simulink model "rtwdemo_pmsmfoc_system_nn"  (Simulink 7.9)
settings: Solver=ode45  SolverMode=SingleTasking  StartTime=0.0  StopTime=0.2  FixedStep=40e-6  RelTol=1e-3
PreLoadFcn:
  | rtwdemo_pmsmfoc_data
StartFcn:
  | clear executionProfile
StopFcn:
  | try
  |   AddExecutionProfileToDataInspector();
  | end
undefined symbols (not defined in the file or in its folder): ctrlConst, DiscIntNeverNeededParam, EnumCommandType, pmsm, sensors, sigbuilder_block
libraries: powerlib x7, simulink x2
Description:
  | Field-Oriented Control of Permanent Magnet Synchronous Machine
  | 
  | Demonstrates a Field-Oriented Control algorithm with Space Vector Modulation for a Permanent Magnet Synchronous Machine (PMSM).
  | The test bench can be used to evaluate the system performance. Examples include turning the motor on, searching for a valid rotor position,
  | transitioning to closed loop operation, and changing speed and torque during closed loop control.
  | The Embedded Processor subsystem contains the controller algorithm (which supports C code generation) as well as simulation models of peripherals.
settings Model: Creator=The MathWorks Inc.  LastModifiedBy=bas  CovMetricSettings=dcmtrzow  CovHTMLOptions=-aTS=1 -bRG=1 -bTC=1 -hTR=0 -nFC=0 -scm=1 -bcm=1 -xEv=0  CovModelRefEnable=off
settings DataIOCC: SaveOutput=off  SaveTime=off
settings OptimizationCC: InlineParams=on  InlineInvariantSignals=on  EnhancedBackFolding=on  StrengthReduction=on  ZeroExternalMemoryAtStartup=off  EfficientFloat2IntCast=on  OptimizeModelRefInitCode=on  LifeSpan=1
settings DebuggingCC: AlgebraicLoopMsg=none  SolverPrmCheckMsg=none  SingleTaskRateTransMsg=error  IntegerOverflowMsg=none  ParameterPrecisionLossMsg=none  UnconnectedInputMsg=none  UnconnectedOutputMsg=none  UnconnectedLineMsg=none  UniqueDataStoreMsg=error  AssertControl=DisableAll
settings HardwareCC: ProdEndianess=LittleEndian  ProdHWDeviceType=Generic->32-bit Embedded Processor
settings ModelReferenceCC: ModelReferenceNumInstancesAllowed=Single
settings RTWCC: SystemTargetFile=nanonote.tlc  TemplateMakefile=nanonote.tmf  Description=Ben NanoNote  GenerateReport=on  RTWVerbose=off  ProcessScript=nanonote_make_rtw_hook  IncludeHyperlinkInReport=on  GenerateTraceInfo=on  GenerateTraceReport=on  GenerateTraceReportSl=on  GenerateTraceReportSf=on  GenerateTraceReportEml=on
settings CodeAppCC: IgnoreCustomStorageClasses=off  IgnoreTestpoints=on  MaxIdLength=64  MATLABFcnDesc=on  CustomSymbolStrGlobalVar=$N$M  CustomSymbolStrType=$N$M  CustomSymbolStrFcn=$N$M$F  CustomSymbolStrFcnArg=$I$N$M  CustomSymbolStrBlkIO=$N$M  CustomSymbolStrMacro=$N$M  MATLABSourceComments=on
settings STFCustomTargetCC: CodeReplacementLibrary=ANSI_C  CombineOutputUpdateFcns=on  ERTCustomFileBanners=on  SupportContinuousTime=off  SupportNonInlinedSFcns=off  GRTInterface=off  SystemTargetFile=nanonote.tlc
settings ERTTargetCC: CodeReplacementLibrary=ANSI_C  MultiwordLength=2048  ParMdlRefBuildCompliant=off  CompOptLevelCompliant=off  ConcurrentExecutionCompliant=off  ERTFirstTimeCompliant=off  ModelStepFunctionPrototypeControlCompliant=off  CPPClassGenCompliant=off  InlinedParameterPlacement=NonHierarchical  ERTCustomFileTemplate=nanonote_srmain.tlc  ConvertIfToSwitch=off  SuppressUnreachableDefaultCases=off
settings CustomProperty: Value=on

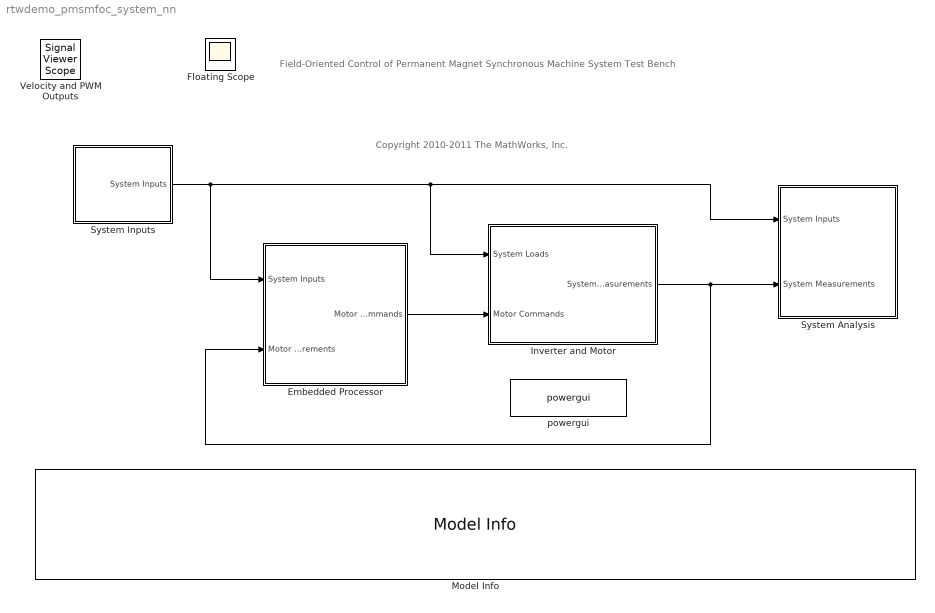
== system rtwdemo_pmsmfoc_system_nn ==
  note: Field-Oriented Control of Permanent Magnet Synchronous Machine
      | System Test Bench
  note: Copyright 2010-2011 The MathWorks, Inc.
  Embedded Processor : Subsystem
      mask Display: image(imread('rtwdemo_pmsmfoc_processor.png'))
  Inverter and Motor : Subsystem  Description=""
      mask Display: image(imread('rtwdemo_pmsmfoc_motor.png'))
  Model Info : simulink/Model-Wide Utilities/Model Info  InitialBlockCM=None  BlockCM=None  Frame=on  DisplayStringWithTags=Model Description: %<Description>  HorizontalTextAlignment=Left  LeftAlignmentValue=0.02  SourceBlockDiagram=rtwdemo_pmsmfoc_system_nn  TagMaxNumber=20
  System Analysis : Subsystem  Description=|
      | System Analysis for Speed Control Design
      | 
      | Analyize and plot signals used to analyize performance of
      | speed  control designs
      mask Display: fprintf('System\nAnalysis')
  System Inputs : Subsystem  Description=""
      mask Display: fprintf('System\nInputs')
  powergui : powerlib/powergui  Priority=1  SimulationMode=Discrete  SolverType=Tustin  SampleTime=1e-005  frequency=60  SPID=off  DisableSnubberDevices=off  DisableRonSwitches=off  DisableVfSwitches=off  SwTol=0  Interpol=off  DisplayEquations=off  FunctionMessages=off  frequencyindice=0  Pbase=100e6  ErrMax=1e-4  Iterations=50  UnitsV=kV  UnitsW=MW  echomessages=off  HookPort=off  EnableUseOfTLC=off  x0status=blocks  RestoreLinks=warning  ResistiveCurrentMeasurement=off  Frange=[0:2:500]  Ylog=off  Xlog=on  ShowGrid=off  save=off  variable=ZData  ZoomFFT=on  StartTime=0.0  cycles=1  DisplayStyle=1  fundamental=60  FreqAxis=off  MaxFrequency=1000  frequencyindicesteady=1  RmsSteady=1  display=off  Ts=0  methode=off
  Floating Scope : Scope
      settings: Floating=on
  Velocity and PWM Outputs : SignalViewerScope  IOType=viewer  NumInputPorts=2  ZoomMode=yonly  RefreshTime=0.035000
      settings: TimeRange=0.14  YMin=-500~0  YMax=4000~3000  SaveName=ScopeData4
  wires:
  Embedded Processor/1(Motor Commands) -> Inverter and Motor/2(Motor Commands)
  Inverter and Motor/1(System Measurements) -> System Analysis/2(System Measurements), Embedded Processor/2(Motor Measurements)
  System Inputs/1(System Inputs) -> System Analysis/1(System Inputs), Inverter and Motor/1(System Loads), Embedded Processor/1(System Inputs)

== system rtwdemo_pmsmfoc_system_nn/Embedded Processor ==
  note: Models hardware on the embedded processor, including
      | the controller algorithm software specification and peripherals.
  note: Embedded Processor
  System Inputs : Inport
  Motor Measurements : Inport  Port=2
  Command Channel : Subsystem  Description=""
      mask Display: fprintf('Command\nChannel')
  Controller Algorithm Software Specification : ModelReference  ModelNameDialog=rtwdemo_pmsmfoc_nn  SimulationMode=Processor-in-the-loop (PIL)  ModelReferenceVersion=1.2950  CopyOfModelName=rtwdemo_pmsmfoc_nn  DefaultDataLogging=on
  Driver Peripherals : Subsystem  Description=""
      mask Display: fprintf('Drivers\nPeripherals')
  Sensor Peripherals : Subsystem  Description=|
      | Elaborate Sensor Models
      | 
      | ADC and QEP and Encoder Models
      mask Display: fprintf('Sensor\nPeripherals')
  Motor Commands : Outport
  wires:
  System Inputs/1 -> Command Channel/1(System Inputs)
  Motor Measurements/1 -> Sensor Peripherals/1(System Measurements)
  Driver Peripherals/1(PWM Duty Cycle) -> Motor Commands/1
  Command Channel/1(motor_on) -> Controller Algorithm Software Specification/1  "motor_on"
  Sensor Peripherals/1(Sensors) -> Controller Algorithm Software Specification/4  "sensors"
  Controller Algorithm Software Specification/1 -> Driver Peripherals/1(pwm_compare)  "pwm_compare"
  Command Channel/2(command_type) -> Controller Algorithm Software Specification/2  "command_type"
  Command Channel/3(command_value) -> Controller Algorithm Software Specification/3  "command_value"
  Controller Algorithm Software Specification/2 -> Driver Peripherals/2(error)  "error"

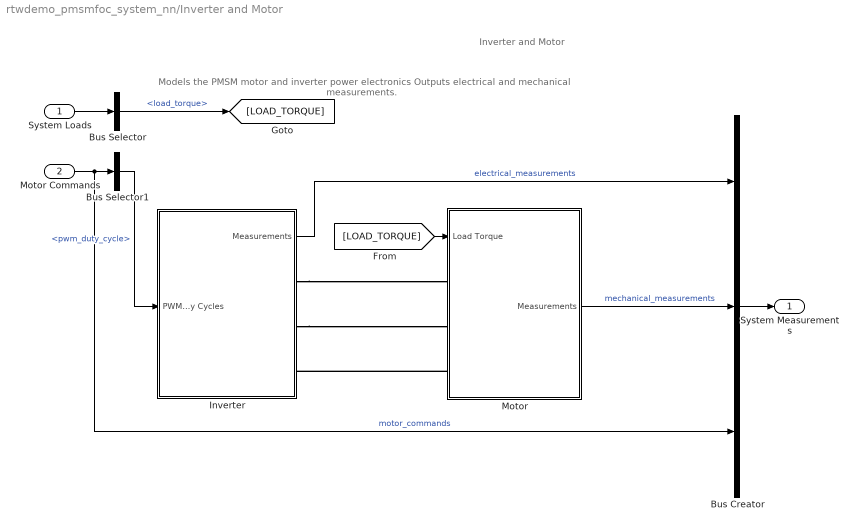
== system rtwdemo_pmsmfoc_system_nn/Inverter and Motor ==
  note: Models the PMSM motor and inverter power electronics
      | Outputs electrical and mechanical measurements.
  note: Inverter and Motor
  System Loads : Inport
  Motor Commands : Inport  Port=2
  Bus Creator : BusCreator  Inputs=3
  Bus Selector : BusSelector  OutputSignals=load_torque
  Bus Selector1 : BusSelector  OutputSignals=pwm_duty_cycle
  Inverter : Subsystem
  Motor : Subsystem
  System Measurements : Outport
  wires:
  Inverter/1(Measurements) -> Bus Creator/1  "electrical_measurements"
  Bus Creator/1 -> System Measurements/1
  Motor/1(Measurements) -> Bus Creator/2  "mechanical_measurements"
  System Loads/1 -> Bus Selector/1
  Motor Commands/1 -> Bus Selector1/1, Bus Creator/3  "motor_commands"
  Bus Selector/1 -> [LOAD_TORQUE]  "<load_torque>"
  Bus Selector1/1 -> Inverter/1(PWM Duty Cycles)  "<pwm_duty_cycle>"
  [LOAD_TORQUE] -> Motor/1(Load Torque)
  connections:
  Inverter/RConn2 -- Motor/LConn2
  Inverter/RConn1 -- Motor/LConn1
  Motor/LConn3 -- Inverter/RConn3

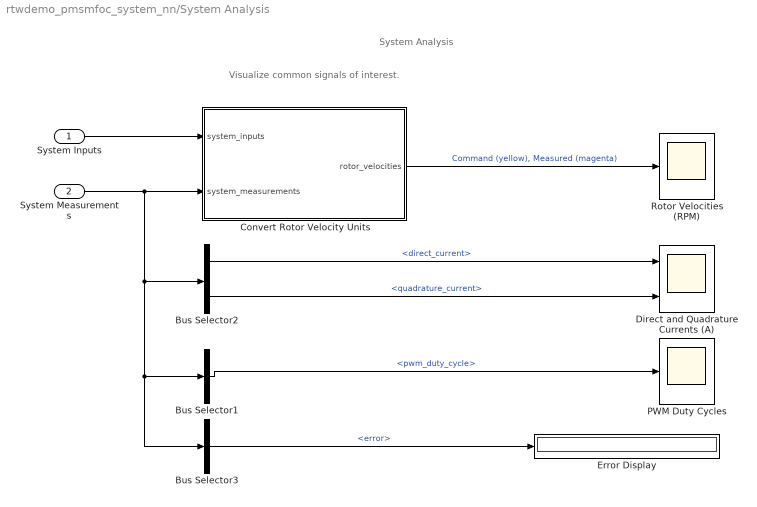
== system rtwdemo_pmsmfoc_system_nn/System Analysis ==
  note: System Analysis
  note: Visualize common signals of interest.
  System Inputs : Inport
  System Measurements : Inport  Port=2
  Bus Selector1 : BusSelector  OutputSignals=motor_commands.pwm_duty_cycle
  Bus Selector2 : BusSelector  OutputSignals=mechanical_measurements.direct_current,mechanical_measurements.quadrature_current
  Bus Selector3 : BusSelector  OutputSignals=motor_commands.error
  Convert Rotor Velocity Units : Subsystem
  Direct and Quadrature Currents (A) : Scope  NumInputPorts=2
      settings: TimeRange=0.2  YMin=-0.04~-0.1  YMax=0.1~0.6000000000000001  SaveName=ScopeData3
  Error Display : Display
  PWM Duty Cycles : Scope
      settings: TimeRange=1.4  YMin=-0.25  YMax=0.25  SaveName=ScopeData2
  Rotor Velocities (RPM) : Scope
      settings: TimeRange=0.2  YMin=-200  YMax=1000
  wires:
  System Measurements/1 -> Convert Rotor Velocity Units/2(system_measurements), Bus Selector3/1, Bus Selector1/1, Bus Selector2/1
  System Inputs/1 -> Convert Rotor Velocity Units/1(system_inputs)
  Convert Rotor Velocity Units/1(rotor_velocities) -> Rotor Velocities (RPM)/1  "Command (yellow), Measured (magenta)"
  Bus Selector1/1 -> PWM Duty Cycles/1  "<pwm_duty_cycle>"
  Bus Selector2/1 -> Direct and Quadrature Currents (A)/1  "<direct_current>"
  Bus Selector2/2 -> Direct and Quadrature Currents (A)/2  "<quadrature_current>"
  Bus Selector3/1 -> Error Display/1  "<error>"

== system rtwdemo_pmsmfoc_system_nn/System Inputs ==
  note: System Inputs
  note: Specify groups of tests in Signal Builder. Outputs are combined into a bus
      | to simplify signal routing through the model.
  Bus Creator : BusCreator
  Command Type : simulink/Sources/Enumerated Constant  OutDataTypeStr=Enum: EnumCommandType  Value=EnumCommandType.Velocity  SampleTime=inf
  Signal Builder Experiments : Subsystem  Tag=STV Subsys  LoadFcn=sigbuilder_block('load');  StartFcn=sigbuilder_block('start');  StopFcn=sigbuilder_block('stop');  ClipboardFcn=sigbuilder_block('clipboard');  mask(Sigbuilder block){}
      mask help: Sigbuilder GUI
      mask init:
      | if ~strcmp(get_param(bdroot(gcbh),'SimulationStatus'),'stopped') tuvar = sigbuilder_block('maskInit'); end
      settings: CopyFcn=sigbuilder_block('copy');  DeleteFcn=sigbuilder_block('delete');  ModelCloseFcn=sigbuilder_block('modelClose');  PreSaveFcn=sigbuilder_block('preSave');  PauseFcn=sigbuilder_block('pause')  ContinueFcn=sigbuilder_block('continue')  NameChangeFcn=sigbuilder_block('namechange');  OpenFcn=sigbuilder_block('open',[64.5 56.25 624.75 441 ]);  CloseFcn=sigbuilder_block('close');
      mask Display: plot(0, 0, 100, 100,[2, 2, 32, 32, 2], [68, 8, 8, 68, 68],[32, 2], [38, 38], [32, 19, 2],[53, 60, 44], [32, 17, 17, 2],[16, 16, 31, 31]);txt = getActiveGroup(gcbh);text(2, 100, txt,'verticalAlignment', 'top');
  oz-in to Newton Meters : Gain  Gain=0.0070615518333
      settings: AttributesFormatString=-------------------------\n%<Gain>
  rpm to rad per sec : Gain  Gain=pi/30
      settings: AttributesFormatString=------------------\n%<Gain>
  System Inputs : Outport
  wires:
  Signal Builder Experiments/3(Load Torque (oz-in)) -> oz-in to Newton Meters/1  "load_torque_ozin"
  Bus Creator/1 -> System Inputs/1
  oz-in to Newton Meters/1 -> Bus Creator/4  "load_torque"
  rpm to rad per sec/1 -> Bus Creator/3  "command"
  Command Type/1 -> Bus Creator/1  "command_type"
  Signal Builder Experiments/1(Motor On (Boolean)) -> Bus Creator/2  "motor_on"
  Signal Builder Experiments/2(Speed Command (RPM)) -> rpm to rad per sec/1  "speed_command_rpm"

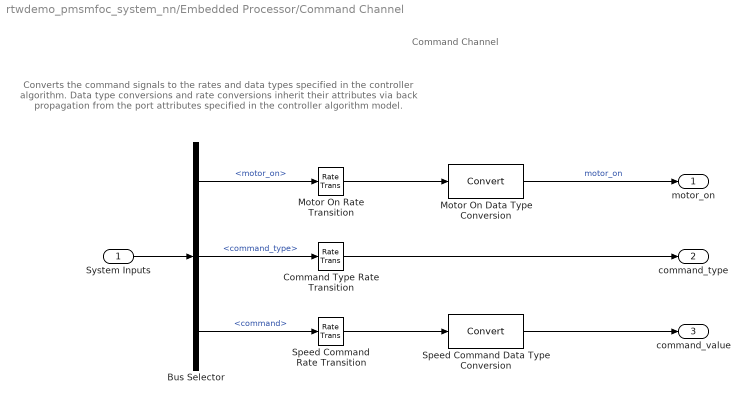
== system rtwdemo_pmsmfoc_system_nn/Embedded Processor/Command Channel ==
  note: Converts the command signals to the rates and data types specified in the controller algorithm.
      | Data type conversions and rate conversions inherit their attributes via back propagation from the
      | port attributes specified in the controller algorithm model.
  note: Command Channel
  System Inputs : Inport
  Bus Selector : BusSelector  OutputSignals=motor_on,command_type,command
  Command Type Rate Transition : RateTransition  Integrity=off  Deterministic=off
  Motor On Data Type Conversion : DataTypeConversion
  Motor On Rate Transition : RateTransition  Integrity=off  Deterministic=off
  Speed Command Data Type Conversion : DataTypeConversion
  Speed Command Rate Transition : RateTransition  Integrity=off  Deterministic=off
  motor_on : Outport
  command_type : Outport  Port=2
  command_value : Outport  Port=3
  wires:
  System Inputs/1 -> Bus Selector/1
  Speed Command Data Type Conversion/1 -> command_value/1
  Bus Selector/1 -> Motor On Rate Transition/1  "<motor_on>"
  Motor On Data Type Conversion/1 -> motor_on/1  "motor_on"
  Motor On Rate Transition/1 -> Motor On Data Type Conversion/1
  Speed Command Rate Transition/1 -> Speed Command Data Type Conversion/1
  Bus Selector/3 -> Speed Command Rate Transition/1  "<command>"
  Bus Selector/2 -> Command Type Rate Transition/1  "<command_type>"
  Command Type Rate Transition/1 -> command_type/1

== system rtwdemo_pmsmfoc_system_nn/Embedded Processor/Driver Peripherals ==
  note: Converts PWM count compare values to a normalized duty cycle.
  note: Driver Peripherals
  pwm_compare : Inport
  error : Inport  Port=2
  Bus Creator : BusCreator  Inputs=2
  Rate Transition : RateTransition  Integrity=off  Deterministic=off  OutPortSampleTime=1e-5
  Units Per PWM Count : Gain  Gain=1 / ctrlConst.PwmCountsPerRevolution  ParamDataTypeStr=double  OutDataTypeStr=double
      settings: AttributesFormatString=------------------------------------------\nGain:\n%<Gain>
  PWM Duty Cycle : Outport
  wires:
  Rate Transition/1 -> Bus Creator/1  "pwm_duty_cycle"
  pwm_compare/1 -> Units Per PWM Count/1
  Units Per PWM Count/1 -> Rate Transition/1
  error/1 -> Bus Creator/2
  Bus Creator/1 -> PWM Duty Cycle/1

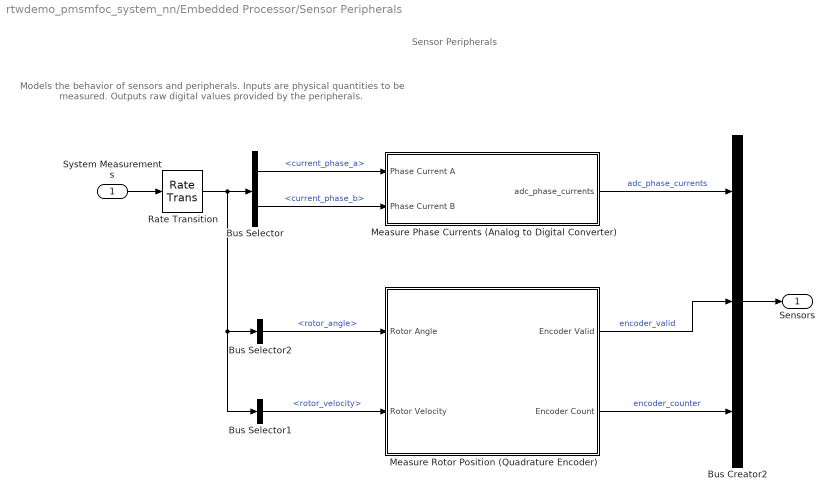
== system rtwdemo_pmsmfoc_system_nn/Embedded Processor/Sensor Peripherals ==
  note: Models the behavior of sensors and peripherals.
      | Inputs are physical quantities to be measured. Outputs raw digital values provided by the peripherals.
  note: Sensor Peripherals
  System Measurements : Inport
  Bus Creator2 : BusCreator  Inputs=3  OutDataTypeStr=Bus: SENSORS_STRUCT
  Bus Selector : BusSelector  OutputSignals=mechanical_measurements.current_phase_a,mechanical_measurements.current_phase_b
  Bus Selector1 : BusSelector  OutputSignals=mechanical_measurements.rotor_velocity
  Bus Selector2 : BusSelector  OutputSignals=mechanical_measurements.rotor_angle
  Measure Phase Currents (Analog to Digital Converter) : Subsystem
  Measure Rotor Position (Quadrature Encoder) : Subsystem
  Rate Transition : RateTransition  OutPortSampleTime=40e-6
  Sensors : Outport
  wires:
  Measure Phase Currents (Analog to Digital Converter)/1(adc_phase_currents) -> Bus Creator2/1  "adc_phase_currents"
  Bus Selector2/1 -> Measure Rotor Position (Quadrature Encoder)/1(Rotor Angle)  "<rotor_angle>"
  Bus Selector1/1 -> Measure Rotor Position (Quadrature Encoder)/2(Rotor Velocity)  "<rotor_velocity>"
  System Measurements/1 -> Rate Transition/1
  Bus Creator2/1 -> Sensors/1
  Measure Rotor Position (Quadrature Encoder)/1(Encoder Valid) -> Bus Creator2/2  "encoder_valid"
  Measure Rotor Position (Quadrature Encoder)/2(Encoder Count) -> Bus Creator2/3  "encoder_counter"
  Bus Selector/1 -> Measure Phase Currents (Analog to Digital Converter)/1(Phase Current A)  "<current_phase_a>"
  Bus Selector/2 -> Measure Phase Currents (Analog to Digital Converter)/2(Phase Current B)  "<current_phase_b>"
  Rate Transition/1 -> Bus Selector1/1, Bus Selector2/1, Bus Selector/1

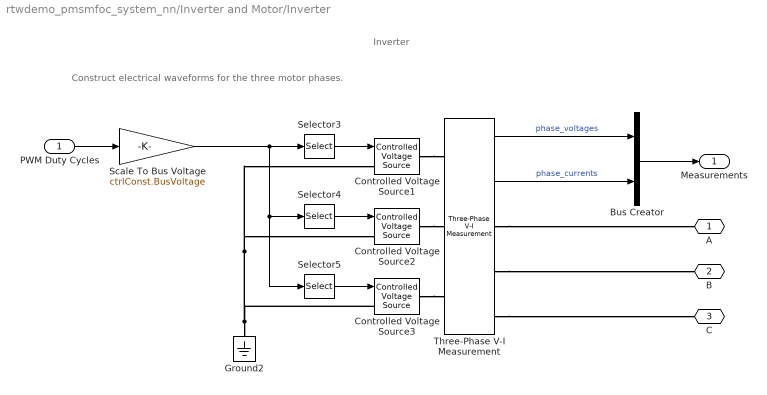
== system rtwdemo_pmsmfoc_system_nn/Inverter and Motor/Inverter ==
  note: Construct electrical waveforms for the three motor phases.
  note: Inverter
  PWM Duty Cycles : Inport
  Bus Creator : BusCreator  Inputs=2
  Controlled Voltage Source1 : powerlib/Electrical Sources/Controlled Voltage Source  Initialize=off  Source_Type=DC  Amplitude=12  Phase=0  Frequency=0  Measurements=None
  Controlled Voltage Source2 : powerlib/Electrical Sources/Controlled Voltage Source  Initialize=off  Source_Type=DC  Amplitude=12  Phase=0  Frequency=0  Measurements=None
  Controlled Voltage Source3 : powerlib/Electrical Sources/Controlled Voltage Source  Initialize=off  Source_Type=DC  Amplitude=12  Phase=0  Frequency=0  Measurements=None
  Ground2 : powerlib/Elements/Ground  LConnTagsString=a
  Scale To Bus Voltage : Gain  Gain=ctrlConst.BusVoltage  ParamDataTypeStr=double  OutDataTypeStr=double
      settings: AttributesFormatString=------------------------------\nGain:\n%<Gain>
  Selector3 : Selector  InputPortWidth=3  IndexOptions=Index vector (dialog)  Indices=[1]  OutputSizes=1
  Selector4 : Selector  InputPortWidth=3  IndexOptions=Index vector (dialog)  Indices=2  OutputSizes=1
  Selector5 : Selector  InputPortWidth=3  IndexOptions=Index vector (dialog)  Indices=3  OutputSizes=1
  Three-Phase V-I Measurement : powerlib/Measurements/Three-Phase V-I Measurement  VoltageMeasurement=phase-to-ground  SetLabelV=off  LabelV=Vabc  Vpu=off  VpuLL=off  CurrentMeasurement=yes  SetLabelI=off  LabelI=Iabc  Ipu=off  Pbase=100e6  Vbase=500e3  OutputType=Complex  PhasorSimulation=off  PSBequivalent=0
  A : PMIOPort  Port=1  Side=Right
  B : PMIOPort  Port=2  Side=Right
  C : PMIOPort  Port=3  Side=Right
  Measurements : Outport
  wires:
  Three-Phase V-I Measurement/2 -> Bus Creator/2  "phase_currents"
  Bus Creator/1 -> Measurements/1
  PWM Duty Cycles/1 -> Scale To Bus Voltage/1
  Three-Phase V-I Measurement/1 -> Bus Creator/1  "phase_voltages"
  Selector3/1 -> Controlled Voltage Source1/1
  Selector4/1 -> Controlled Voltage Source2/1
  Selector5/1 -> Controlled Voltage Source3/1
  Scale To Bus Voltage/1 -> Selector3/1, Selector5/1, Selector4/1
  connections:
  Three-Phase V-I Measurement/RConn1 -- A/RConn1
  Three-Phase V-I Measurement/RConn2 -- B/RConn1
  Three-Phase V-I Measurement/RConn3 -- C/RConn1
  Ground2/LConn1 -- Controlled Voltage Source3/LConn1 -- Controlled Voltage Source1/LConn1 -- Controlled Voltage Source2/LConn1
  Controlled Voltage Source2/RConn1 -- Three-Phase V-I Measurement/LConn2
  Controlled Voltage Source1/RConn1 -- Three-Phase V-I Measurement/LConn1
  Controlled Voltage Source3/RConn1 -- Three-Phase V-I Measurement/LConn3

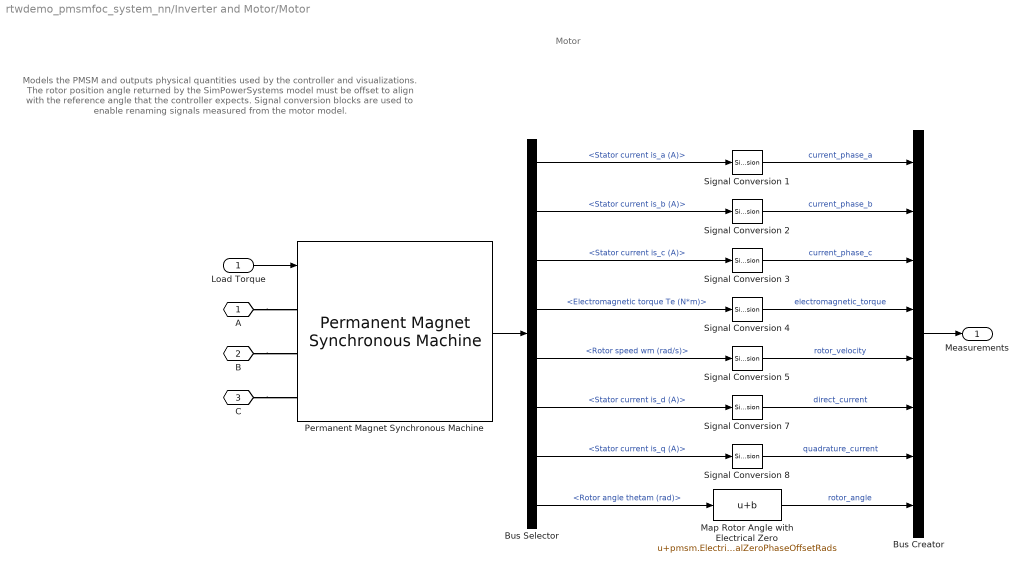
== system rtwdemo_pmsmfoc_system_nn/Inverter and Motor/Motor ==
  note: Motor
  note: Models the PMSM and outputs physical quantities used by the controller and visualizations.
      | The rotor position angle returned by the SimPowerSystems model must be offset to align with the reference angle that the controller expects.
      | Signal conversion blocks are used to enable renaming signals measured from the motor model.
  Load Torque : Inport
  Bus Creator : BusCreator  Inputs=8
  Bus Selector : BusSelector  OutputSignals=Stator current is_a (A),Stator current is_b (A),Stator current is_c (A),Electromagnetic torque Te (N*m),Rotor speed wm (rad/s),Stator current is_d (A),Stator current is_q (A),Rotor angle thetam (rad)
  Map Rotor Angle with Electrical Zero : Bias  Bias=pmsm.ElectricalZeroPhaseOffsetRads
      settings: AttributesFormatString=----------------------------------------\n%<Bias>
  Permanent Magnet Synchronous Machine : powerlib/Machines/Permanent Magnet Synchronous Machine  NbPhases=3  FluxDistribution=Sinusoidal  RotorType=Salient-pole  MechanicalLoad=Torque Tm  PresetModel=No  ShowDetailedParameters=on  Resistance=pmsm.StatorPhaseResistance  Inductance=8.5e-3  dqInductances=[pmsm.InductanceLd pmsm.InductanceLq]  La=0.000835  MachineConstant=Torque Constant (N.m / A_peak)  Flux=0.0058847  VoltageCst=4.2694  TorqueCst=pmsm.TorqueConstant  Flat=120  Mechanical=[pmsm.Inertia, pmsm.ViscousDamping, pmsm.PolePairs, pmsm.StaticFriction]  PolePairs=4  InitialConditions=[0, pmsm.ThetaInitDegrees, 0, 0]  InitialConditions5ph=[0 0 0 0 0 0]  TsPowergui=0  TsBlock=-1  RefAngle=90 degrees behind phase A axis (modified Park)
  Signal Conversion {1..5,7..8} (7 alike) : SignalConversion  ConversionOutput=Contiguous copy
  A : PMIOPort  Port=1  Side=Left
  B : PMIOPort  Port=2  Side=Left
  C : PMIOPort  Port=3  Side=Left
  Measurements : Outport
  wires:
  Permanent Magnet Synchronous Machine/1 -> Bus Selector/1
  Load Torque/1 -> Permanent Magnet Synchronous Machine/1
  Bus Selector/1 -> Signal Conversion 1/1  "<Stator current is_a (A)>"
  Bus Selector/2 -> Signal Conversion 2/1  "<Stator current is_b (A)>"
  Bus Selector/3 -> Signal Conversion 3/1  "<Stator current is_c (A)>"
  Bus Selector/5 -> Signal Conversion 5/1  "<Rotor speed wm (rad/s)>"
  Bus Selector/4 -> Signal Conversion 4/1  "<Electromagnetic torque Te (N*m)>"
  Bus Creator/1 -> Measurements/1
  Signal Conversion 1/1 -> Bus Creator/1  "current_phase_a"
  Signal Conversion 2/1 -> Bus Creator/2  "current_phase_b"
  Signal Conversion 3/1 -> Bus Creator/3  "current_phase_c"
  Signal Conversion 4/1 -> Bus Creator/4  "electromagnetic_torque"
  Signal Conversion 5/1 -> Bus Creator/5  "rotor_velocity"
  Bus Selector/8 -> Map Rotor Angle with Electrical Zero/1  "<Rotor angle thetam (rad)>"
  Signal Conversion 7/1 -> Bus Creator/6  "direct_current"
  Signal Conversion 8/1 -> Bus Creator/7  "quadrature_current"
  Map Rotor Angle with Electrical Zero/1 -> Bus Creator/8  "rotor_angle"
  Bus Selector/6 -> Signal Conversion 7/1  "<Stator current is_d (A)>"
  Bus Selector/7 -> Signal Conversion 8/1  "<Stator current is_q (A)>"
  connections:
  A/RConn1 -- Permanent Magnet Synchronous Machine/LConn1
  B/RConn1 -- Permanent Magnet Synchronous Machine/LConn2
  C/RConn1 -- Permanent Magnet Synchronous Machine/LConn3

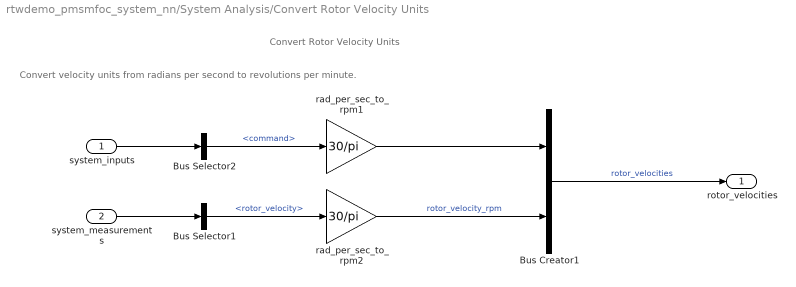
== system rtwdemo_pmsmfoc_system_nn/System Analysis/Convert Rotor Velocity Units ==
  note: Convert Rotor Velocity Units
  note: Convert velocity units from radians per second to revolutions per minute.
  system_inputs : Inport
  system_measurements : Inport  Port=2
  Bus Creator1 : BusCreator  Inputs=2
  Bus Selector1 : BusSelector  OutputSignals=mechanical_measurements.rotor_velocity
  Bus Selector2 : BusSelector  OutputSignals=command
  rad_per_sec_to_rpm1 : Gain  Gain=30/pi
  rad_per_sec_to_rpm2 : Gain  Gain=30/pi
  rotor_velocities : Outport
  wires:
  Bus Selector2/1 -> rad_per_sec_to_rpm1/1  "<command>"
  Bus Selector1/1 -> rad_per_sec_to_rpm2/1  "<rotor_velocity>"
  Bus Creator1/1 -> rotor_velocities/1  "rotor_velocities"
  system_inputs/1 -> Bus Selector2/1
  system_measurements/1 -> Bus Selector1/1
  rad_per_sec_to_rpm1/1 -> Bus Creator1/1
  rad_per_sec_to_rpm2/1 -> Bus Creator1/2  "rotor_velocity_rpm"

== system rtwdemo_pmsmfoc_system_nn/System Inputs/Signal Builder Experiments ==
  Demux : Demux  Tag=STV Demux  Outputs=3
  FromWs : FromWorkspace  Tag=STV FromWs  VariableName=tuvar  SampleTime=1e-5  OutputAfterFinalValue=Holding final value  SigBuilderData=DataTag0  VnvData=DataTag1
      SigBuilderData=|
      | common.afterFinalStr = 'Hold final value'
      | common.sampleTime = '1e-5'
      | dataSet(1).timeRange = [0 0.16]
      | dataSet(1).name = 'No Load Velocity Control'
      | dataSet(2).timeRange = [0 0.16]
      | dataSet(2).name = 'Velocity On/Off'
      | dataSet(3).timeRange = [0 0.16]
      | dataSet(3).name = 'Torque Step'
      | dataSet(4).timeRange = [0 0.14]
      | dataSet(4).name = 'Hi Velocity'
      | dataSet(5).timeRange = [0 0.16]
      | dataSet(5).name = 'Velocity Step Validation'
      | dataSet(6).timeRange = [0 0.2]
      | dataSet(6).name = 'Hi Velocity On/Off'
      | sbobj.Groups(1).Name = 'No Load Velocity Control'
      | sbobj.Groups(1).Signals(1).Name = 'Motor On (Boolean)'
      | sbobj.Groups(1).Signals(1).XData = [0 0.01 0.01 0.16]
      | sbobj.Groups(1).Signals(1).YData = [0 0 1 1]
      | sbobj.Groups(1).Signals(2).Name = 'Speed Command (RPM)'
      | sbobj.Groups(1).Signals(2).XData = [0 0.16]
      | sbobj.Groups(1).Signals(2).YData = [1000 1000]
      | sbobj.Groups(1).Signals(3).Name = 'Load Torque (oz-in)'
      | sbobj.Groups(1).Signals(3).XData = [0 0.16]
      | sbobj.Groups(1).Signals(3).YData = [0 0]
      | sbobj.Groups(1).TimeRange = [0 0.16]
      | sbobj.Groups(2).Name = 'Velocity On/Off'
      | sbobj.Groups(2).Signals(1).Name = 'Motor On (Boolean)'
      | sbobj.Groups(2).Signals(1).XData = [0 0.01 0.01 0.065 0.065 0.16]
      | sbobj.Groups(2).Signals(1).YData = [0 0 1 1 0 0]
      | sbobj.Groups(2).Signals(2).Name = 'Speed Command (RPM)'
      | sbobj.Groups(2).Signals(2).XData = [0 0.16]
      | sbobj.Groups(2).Signals(2).YData = [1000 1000]
      | sbobj.Groups(2).Signals(3).Name = 'Load Torque (oz-in)'
      | sbobj.Groups(2).Signals(3).XData = [0 0.16]
      | sbobj.Groups(2).Signals(3).YData = [0.3 0.3]
      | sbobj.Groups(2).TimeRange = [0 0.16]
      | sbobj.Groups(3).Name = 'Torque Step'
      | sbobj.Groups(3).Signals(1).Name = 'Motor On (Boolean)'
      | sbobj.Groups(3).Signals(1).XData = [0 0.16]
      | sbobj.Groups(3).Signals(1).YData = [1 1]
      | sbobj.Groups(3).Signals(2).Name = 'Speed Command (RPM)'
      | sbobj.Groups(3).Signals(2).XData = [0 0.16]
      | sbobj.Groups(3).Signals(2).YData = [1000 1000]
      | sbobj.Groups(3).Signals(3).Name = 'Load Torque (oz-in)'
      | sbobj.Groups(3).Signals(3).XData = [0 0.02 0.02 0.16]
      | sbobj.Groups(3).Signals(3).YData = [0 0 0.2 0.2]
      | sbobj.Groups(3).TimeRange = [0 0.16]
      | sbobj.Groups(4).Name = 'Hi Velocity'
      | sbobj.Groups(4).Signals(1).Name = 'Motor On (Boolean)'
      | sbobj.Groups(4).Signals(1).XData = [0 0.01 0.01 0.14]
      | sbobj.Groups(4).Signals(1).YData = [0 0 1 1]
      | sbobj.Groups(4).Signals(2).Name = 'Speed Command (RPM)'
      | sbobj.Groups(4).Signals(2).XData = [0 0.14]
      | sbobj.Groups(4).Signals(2).YData = [4000 4000]
      | sbobj.Groups(4).Signals(3).Name = 'Load Torque (oz-in)'
      | sbobj.Groups(4).Signals(3).XData = [0 0.14]
      | sbobj.Groups(4).Signals(3).YData = [0 0]
      | sbobj.Groups(4).TimeRange = [0 0.14]
      | sbobj.Groups(5).Name = 'Velocity Step Validation'
      | sbobj.Groups(5).Signals(1).Name = 'Motor On (Boolean)'
      | sbobj.Groups(5).Signals(1).XData = [0 0.015 0.015 0.16]
      | sbobj.Groups(5).Signals(1).YData = [0 0 1 1]
      | sbobj.Groups(5).Signals(2).Name = 'Speed Command (RPM)'
      | sbobj.Groups(5).Signals(2).XData = [0 0.16]
      | sbobj.Groups(5).Signals(2).YData = [954.929658551 954.929658551]
      | sbobj.Groups(5).Signals(3).Name = 'Load Torque (oz-in)'
      | sbobj.Groups(5).Signals(3).XData = [0 0.16]
      | sbobj.Groups(5).Signals(3).YData = [0 0]
      | sbobj.Groups(5).TimeRange = [0 0.16]
      | sbobj.Groups(6).Name = 'Hi Velocity On/Off'
      | sbobj.Groups(6).Signals(1).Name = 'Motor On (Boolean)'
      | sbobj.Groups(6).Signals(1).XData = [0 0.01 0.01 0.18 0.18 0.2]
      | sbobj.Groups(6).Signals(1).YData = [0 0 1 1 0 0]
      | sbobj.Groups(6).Signals(2).Name = 'Speed Command (RPM)'
      | sbobj.Groups(6).Signals(2).XData = [0 0.2]
      | sbobj.Groups(6).Signals(2).YData = [4000 4000]
      | sbobj.Groups(6).Signals(3).Name = 'Load Torque (oz-in)'
      | sbobj.Groups(6).Signals(3).XData = [0 0.2]
      | sbobj.Groups(6).Signals(3).YData = [0 0]
      | sbobj.Groups(6).TimeRange = [0 0.2]
  Motor On (Boolean) : Outport  Tag=STV Outport
  Speed Command (RPM) : Outport  Tag=STV Outport  Port=2
  Load Torque (oz-in) : Outport  Tag=STV Outport  Port=3
  wires:
  FromWs/1 -> Demux/1
  Demux/1 -> Motor On (Boolean)/1
  Demux/2 -> Speed Command (RPM)/1
  Demux/3 -> Load Torque (oz-in)/1

== system rtwdemo_pmsmfoc_system_nn/Embedded Processor/Sensor Peripherals/Measure Phase Currents (Analog to Digital Converter) ==
  note: Models the behavior of the current sensor and analog to digital voltage conversion.
  note: Measure Phase Currents
      | (Analog to Digital Converter)
  Phase Current A : Inport
  Phase Current B : Inport  Port=2
  Current Sensor : Subsystem
  Driver Noise : Subsystem
      mask init:
      | if evalin('base','sensors.ADC.NoiseEnable')
      |     enable = 'Enabled';
      | else
      |     enable = 'Disabled';
      | end
      mask Display: fprintf(['ADC Driver Noise\n(' enable ')'])
  Vector Concatenate : Concatenate
  adc_phase_currents : Outport
  wires:
  Current Sensor/1(Driver Units) -> Driver Noise/1(In)
  Vector Concatenate/1 -> Current Sensor/1(Phase Currents)
  Driver Noise/1(Out) -> adc_phase_currents/1
  Phase Current A/1 -> Vector Concatenate/1
  Phase Current B/1 -> Vector Concatenate/2

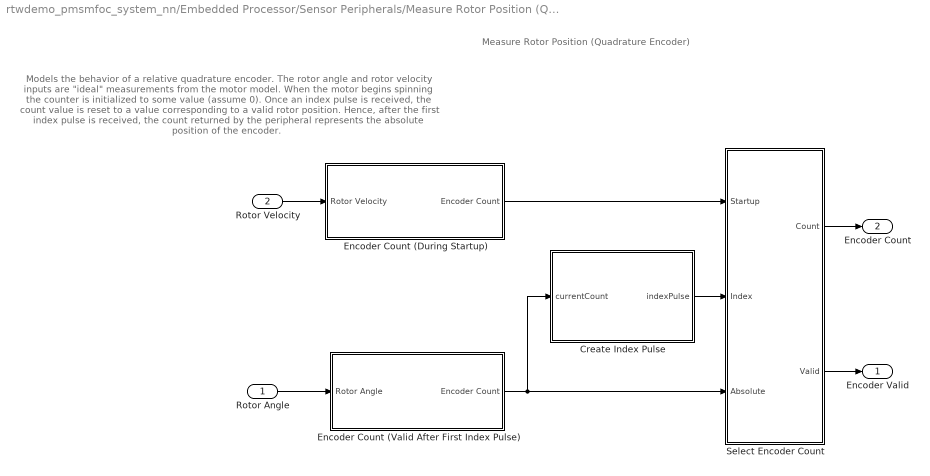
== system rtwdemo_pmsmfoc_system_nn/Embedded Processor/Sensor Peripherals/Measure Rotor Position (Quadrature Encoder) ==
  note: Models the behavior of a relative quadrature encoder. The rotor angle and rotor velocity inputs are "ideal" measurements from the motor model.
      | When the motor begins spinning the counter is initialized to some value (assume 0).
      | Once an index pulse is received, the count value is reset to a value corresponding to a valid rotor position.
      | Hence, after the first index pulse is received, the count returned by the peripheral represents the absolute position of the encoder.
  note: Measure Rotor Position
      | (Quadrature Encoder)
  Rotor Angle : Inport
  Rotor Velocity : Inport  Port=2
  Create Index Pulse : MATLAB Function  TreatAsAtomicUnit=on
  Encoder Count (During Startup) : Subsystem
  Encoder Count (Valid After First Index Pulse) : Subsystem
  Select Encoder Count : Subsystem
  Encoder Valid : Outport
  Encoder Count : Outport  Port=2
  wires:
  Select Encoder Count/1(Count) -> Encoder Count/1
  Create Index Pulse/1(indexPulse) -> Select Encoder Count/2(Index)
  Encoder Count (Valid After First Index Pulse)/1(Encoder Count) -> Select Encoder Count/3(Absolute), Create Index Pulse/1(currentCount)
  Encoder Count (During Startup)/1(Encoder Count) -> Select Encoder Count/1(Startup)
  Rotor Velocity/1 -> Encoder Count (During Startup)/1(Rotor Velocity)
  Rotor Angle/1 -> Encoder Count (Valid After First Index Pulse)/1(Rotor Angle)
  Select Encoder Count/2(Valid) -> Encoder Valid/1

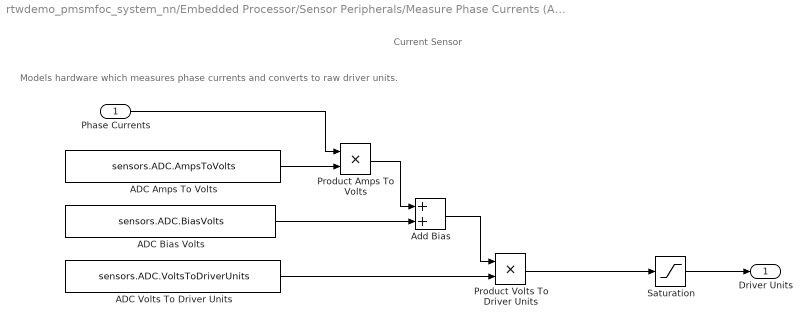
== system rtwdemo_pmsmfoc_system_nn/Embedded Processor/Sensor Peripherals/Measure Phase Currents (Analog to Digital Converter)/Current Sensor ==
  note: Current Sensor
  note: Models hardware which measures phase currents and converts to raw driver units.
  Phase Currents : Inport
  ADC Amps To Volts : Constant  Value=sensors.ADC.AmpsToVolts
  ADC Bias Volts : Constant  Value=sensors.ADC.BiasVolts
  ADC Volts To Driver Units : Constant  Value=sensors.ADC.VoltsToDriverUnits
  Add Bias : Sum
  Product Amps To Volts : Product  RndMeth=Zero
  Product Volts To Driver Units : Product  RndMeth=Zero
  Saturation : Saturate  UpperLimit=sensors.ADC.MaxDriverUnits  LowerLimit=0  OutDataTypeStr=uint16
      settings: AttributesFormatString=----------------------------\nUpper Limit: %<UpperLimit>\nLower Limit: %<LowerLimit>
  Driver Units : Outport
  wires:
  Phase Currents/1 -> Product Amps To Volts/1
  ADC Amps To Volts/1 -> Product Amps To Volts/2
  Product Amps To Volts/1 -> Add Bias/1
  ADC Bias Volts/1 -> Add Bias/2
  Add Bias/1 -> Product Volts To Driver Units/1
  ADC Volts To Driver Units/1 -> Product Volts To Driver Units/2
  Product Volts To Driver Units/1 -> Saturation/1
  Saturation/1 -> Driver Units/1

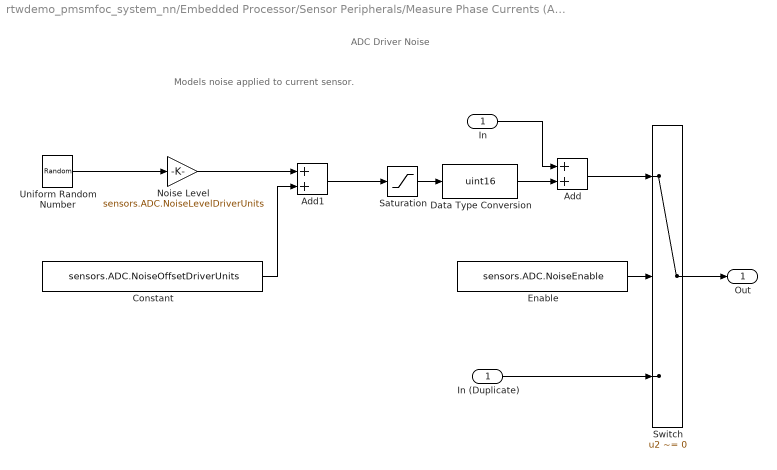
== system rtwdemo_pmsmfoc_system_nn/Embedded Processor/Sensor Peripherals/Measure Phase Currents (Analog to Digital Converter)/Driver Noise ==
  note: ADC Driver Noise
  note: Models noise applied to current sensor.
  In : Inport
  Add : Sum  RndMeth=Convergent  SaturateOnIntegerOverflow=on
  Add1 : Sum  RndMeth=Convergent  SaturateOnIntegerOverflow=on
  Constant : Constant  Value=sensors.ADC.NoiseOffsetDriverUnits
  Data Type Conversion : DataTypeConversion  OutDataTypeStr=uint16  RndMeth=Convergent
  Enable : Constant  Value=sensors.ADC.NoiseEnable
  In (Duplicate) : InportShadow  Port=1
  Noise Level : Gain  Gain=sensors.ADC.NoiseLevelDriverUnits
      settings: AttributesFormatString=------------------------------------\n%<Gain>
  Saturation : Saturate  UpperLimit=sensors.ADC.MaxDriverUnits  LowerLimit=0  OutDataTypeStr=uint16
      settings: AttributesFormatString=----------------------------\nUpper Limit: %<UpperLimit>\nLower Limit: %<LowerLimit>
  Switch : Switch  Criteria=u2 ~= 0
  Uniform Random Number : UniformRandomNumber  Minimum=[0 0]  Maximum=[1 1]  SampleTime=ctrlConst.TsHi
  Out : Outport
  wires:
  Switch/1 -> Out/1
  Uniform Random Number/1 -> Noise Level/1
  Noise Level/1 -> Add1/1
  Constant/1 -> Add1/2
  Add1/1 -> Saturation/1
  Saturation/1 -> Data Type Conversion/1
  Add/1 -> Switch/1
  In/1 -> Add/1
  Data Type Conversion/1 -> Add/2
  In (Duplicate)/1 -> Switch/3
  Enable/1 -> Switch/2

== system rtwdemo_pmsmfoc_system_nn/Embedded Processor/Sensor Peripherals/Measure Rotor Position (Quadrature Encoder)/Encoder Count (During Startup) ==
  note: Approximate the count value provided by the encoder peripheral during startup (before reaching the first index pulse).
      | The pulse train generated by the encoder is not modeled.
  note: Encoder Count
      | (During Startup)
  Rotor Velocity : Inport
  Counts per Radian : Gain  Gain=ctrlConst.EncoderCountsPerRevolution/(2*pi)
      settings: AttributesFormatString=--------------------------------------------------\nGain:\n%<Gain>
  Discrete-Time Integrator : DiscreteIntegrator  InitialCondition=sensors.Encoder.InitialAngleRads  SampleTime=-1  ICPrevOutput=DiscIntNeverNeededParam  ICPrevScaledInput=DiscIntNeverNeededParam
      settings: AttributesFormatString=------------------------------\nInitial Condition: %<InitialCondition>
  Encoder Angle Data Type : DataTypeConversion  OutDataTypeStr=uint16
  Math Function : Math  Operator=mod  SaturateOnIntegerOverflow=on
  Radians Per Cycle : Constant  Value=2*pi
  Encoder Count : Outport
  wires:
  Radians Per Cycle/1 -> Math Function/2
  Math Function/1 -> Counts per Radian/1
  Counts per Radian/1 -> Encoder Angle Data Type/1
  Rotor Velocity/1 -> Discrete-Time Integrator/1
  Encoder Angle Data Type/1 -> Encoder Count/1
  Discrete-Time Integrator/1 -> Math Function/1

== system rtwdemo_pmsmfoc_system_nn/Embedded Processor/Sensor Peripherals/Measure Rotor Position (Quadrature Encoder)/Encoder Count (Valid After First Index Pulse) ==
  note: Encoder Count
      | (Valid After First Index Pulse)
  note: Model the count value provided by the encoder when the absolute position is known.
      | The absolute position is known after reaching the first index pulse.
      | The pulse train generated by the encoder is not modeled.
  Rotor Angle : Inport
  Add : Sum
  Counts per Radian : Gain  Gain=ctrlConst.EncoderCountsPerRevolution/(2*pi)
      settings: AttributesFormatString=-------------------------------------------\nGain:\n%<Gain>
  Encoder Angle Data Type : DataTypeConversion  OutDataTypeStr=uint16
  Math Function : Math  Operator=mod  SaturateOnIntegerOverflow=on
  Offset_Between_Mechanical_Zero_And_Encoder_Zero : Constant  Value=sensors.Encoder.MechanicalToEncoderZeroOffsetRads
  Radians Per Cycle : Constant  Value=2*pi
  Encoder Count : Outport
  wires:
  Encoder Angle Data Type/1 -> Encoder Count/1
  Counts per Radian/1 -> Encoder Angle Data Type/1
  Radians Per Cycle/1 -> Math Function/2
  Offset_Between_Mechanical_Zero_And_Encoder_Zero/1 -> Add/2
  Math Function/1 -> Counts per Radian/1
  Rotor Angle/1 -> Add/1
  Add/1 -> Math Function/1

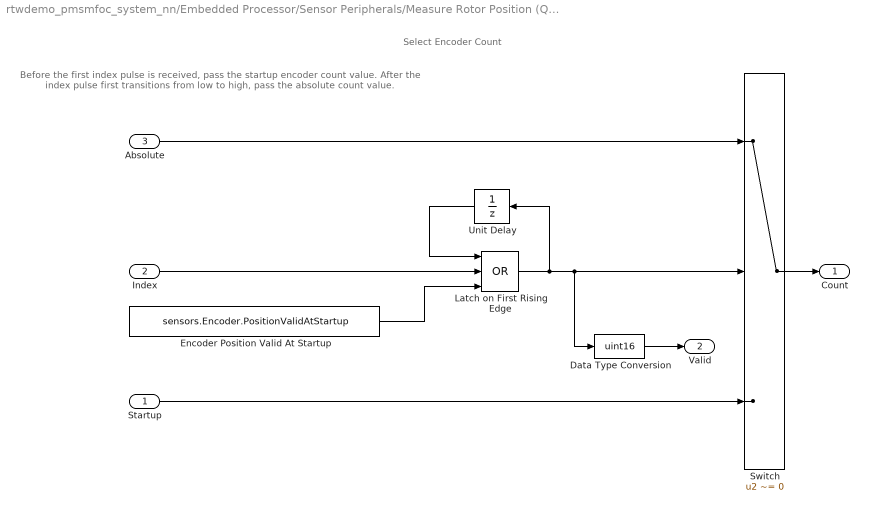
== system rtwdemo_pmsmfoc_system_nn/Embedded Processor/Sensor Peripherals/Measure Rotor Position (Quadrature Encoder)/Select Encoder Count ==
  note: Select Encoder Count
  note: Before the first index pulse is received, pass the startup encoder count value.
      | After the index pulse first transitions from low to high, pass the absolute count value.
  Startup : Inport
  Index : Inport  Port=2
  Absolute : Inport  Port=3
  Data Type Conversion : DataTypeConversion  OutDataTypeStr=uint16
  Encoder Position Valid At Startup : Constant  Value=sensors.Encoder.PositionValidAtStartup
  Latch on First Rising Edge : Logic  Operator=OR  Inputs=3  IconShape=distinctive  AllPortsSameDT=off  OutDataTypeStr=boolean
  Switch : Switch  Criteria=u2 ~= 0
  Unit Delay : UnitDelay  SampleTime=-1
  Count : Outport
  Valid : Outport  Port=2
  wires:
  Latch on First Rising Edge/1 -> Unit Delay/1, Switch/2, Data Type Conversion/1
  Absolute/1 -> Switch/1
  Switch/1 -> Count/1
  Startup/1 -> Switch/3
  Unit Delay/1 -> Latch on First Rising Edge/1
  Index/1 -> Latch on First Rising Edge/2
  Encoder Position Valid At Startup/1 -> Latch on First Rising Edge/3
  Data Type Conversion/1 -> Valid/1

== matlab function Embedded Processor/Sensor Peripherals/Measure Rotor Position (Quadrature Encoder)/Create Index Pulse ==
  data: currentCount input double; indexPulse output double size=1; ctrlConst parameter double
function indexPulse = fcn( currentCount, ctrlConst )  %#codegen
% Create an index pulse at position 2pi

    persistent previousCount;

    if isempty(previousCount)
        previousCount = currentCount;
    end

    % Detect the wrap. Assumes simulation will not allow moving pi rads
    % in one simulation step
    if abs(double(currentCount) - double(previousCount)) > (ctrlConst.EncoderCountsPerRevolution/2)
        index = true;
    else
        index = false;
    end

    previousCount = currentCount;

    indexPulse = uint16(index);
end
